simulink model "pyle_tf"  (R2020a)
settings: Solver=VariableStepAuto  StartTime=0.0  StopTime=0.2  RelTol=1e-3
libraries: fl_lib x71, nesl_utility x17, simulink x5, powerlib_meascontrol x1, ee_lib x1
(part 2 of 2)

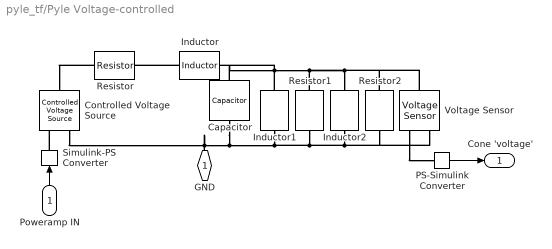
== system pyle_tf/Pyle Voltage-controlled ==
  Poweramp IN : Inport
  Capacitor : fl_lib/Electrical/Electrical Elements/Capacitor  c=388.95 uF  r=0 Ohm  g=0 1/Ohm  i_specify=off  i_priority=None  i=0 A  i_nominal_specify=off  i_nominal_unit=A  i_nominal_value=1  v_specify=off  v_priority=None  v=0 V  v_nominal_specify=off  v_nominal_unit=V  v_nominal_value=1  vc_specify=off  vc_priority=High  vc=0 V  vc_nominal_specify=off  vc_nominal_unit=V  vc_nominal_value=1
  Controlled Voltage Source : fl_lib/Electrical/Electrical Sources/Controlled Voltage Source
  Inductor : fl_lib/Electrical/Electrical Elements/Inductor  l=148.8 uH  r=0 Ohm  g=0 1/Ohm  i_specify=off  i_priority=None  i=0 A  i_nominal_specify=off  i_nominal_unit=A  i_nominal_value=1  v_specify=off  v_priority=None  v=0 V  v_nominal_specify=off  v_nominal_unit=V  v_nominal_value=1  i_L_specify=off  i_L_priority=High  i_L=0 A  i_L_nominal_specify=off  i_L_nominal_unit=A  i_L_nominal_value=1
  Inductor1 : fl_lib/Electrical/Electrical Elements/Inductor  l=23.9 mH  r=0 Ohm  g=0 1/Ohm  i_specify=off  i_priority=None  i=0 A  i_nominal_specify=off  i_nominal_unit=A  i_nominal_value=1  v_specify=off  v_priority=None  v=0 V  v_nominal_specify=off  v_nominal_unit=V  v_nominal_value=1  i_L_specify=off  i_L_priority=High  i_L=0 A  i_L_nominal_specify=off  i_L_nominal_unit=A  i_L_nominal_value=1
  Inductor2 : fl_lib/Electrical/Electrical Elements/Inductor  l=9 mH  r=0 Ohm  g=0 1/Ohm  i_specify=off  i_priority=None  i=0 A  i_nominal_specify=off  i_nominal_unit=A  i_nominal_value=1  v_specify=off  v_priority=None  v=0 V  v_nominal_specify=off  v_nominal_unit=V  v_nominal_value=1  i_L_specify=off  i_L_priority=High  i_L=0 A  i_L_nominal_specify=off  i_L_nominal_unit=A  i_L_nominal_value=1
  PS-Simulink Converter : nesl_utility/PS-Simulink Converter  PhysicalDomain=network_engine_domain  SubClassName=ps_output  LeftPortType=input  RightPortType=output  PseudoPeriodic=off  Frequencies=[]  Unit=inherit  AffineConversion=off
  Resistor : fl_lib/Electrical/Electrical Elements/Resistor  R=3.4 Ohm  i_specify=off  i_priority=None  i=0 A  i_nominal_specify=off  i_nominal_unit=A  i_nominal_value=1  v_specify=off  v_priority=None  v=0 V  v_nominal_specify=off  v_nominal_unit=V  v_nominal_value=1
  Resistor1 : fl_lib/Electrical/Electrical Elements/Resistor  R=28.42 Ohm  i_specify=off  i_priority=None  i=0 A  i_nominal_specify=off  i_nominal_unit=A  i_nominal_value=1  v_specify=off  v_priority=None  v=0 V  v_nominal_specify=off  v_nominal_unit=V  v_nominal_value=1
  Resistor2 : fl_lib/Electrical/Electrical Elements/Resistor  R=282 Ohm  i_specify=off  i_priority=None  i=0 A  i_nominal_specify=off  i_nominal_unit=A  i_nominal_value=1  v_specify=off  v_priority=None  v=0 V  v_nominal_specify=off  v_nominal_unit=V  v_nominal_value=1
  Simulink-PS Converter : nesl_utility/Simulink-PS Converter  PhysicalDomain=network_engine_domain  SubClassName=ps_input  LeftPortType=input  RightPortType=output  PseudoPeriodic=off  Frequencies=[]  NoiseDistribution=none  NoiseParameters=[]  Unit=1  AffineConversion=off  FilteringAndDerivatives=provide  SimscapeFilterOrder=1  InputFilterTimeConstant=0.001  UdotUserProvided=0
  Voltage Sensor : fl_lib/Electrical/Electrical Sensors/Voltage Sensor
  GND : PMIOPort  Side=Right
  Cone 'voltage' : Outport
  wires:
  PS-Simulink Converter/1 -> Cone 'voltage'/1
  Poweramp IN/1 -> Simulink-PS Converter/1
  connections:
  Voltage Sensor/RConn1 -- PS-Simulink Converter/LConn1
  Simulink-PS Converter/RConn1 -- Controlled Voltage Source/RConn1
  Controlled Voltage Source/RConn2 -- GND/RConn1 -- Resistor2/RConn1 -- Voltage Sensor/RConn2 -- Inductor2/RConn1 -- Resistor1/RConn1 -- Inductor1/RConn1 -- Capacitor/RConn1
  Inductor1/LConn1 -- Inductor2/LConn1 -- Voltage Sensor/LConn1 -- Resistor2/LConn1 -- Resistor1/LConn1 -- Capacitor/LConn1 -- Inductor/RConn1
  Inductor/LConn1 -- Resistor/RConn1
  Resistor/LConn1 -- Controlled Voltage Source/LConn1

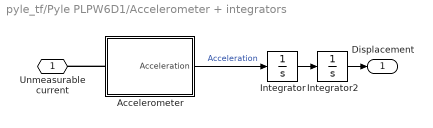
== system pyle_tf/Pyle PLPW6D1/Accelerometer + integrators ==
  Accelerometer : Subsystem
  Integrator : Integrator
  Integrator2 : Integrator
  Unmeasurable current : PMIOPort  Side=Left
  Displacement : Outport
  wires:
  Integrator2/1 -> Displacement/1
  Integrator/1 -> Integrator2/1
  Accelerometer/1(Acceleration) -> Integrator/1  "Acceleration"
  connections:
  Accelerometer/LConn1 -- Unmeasurable current/RConn1

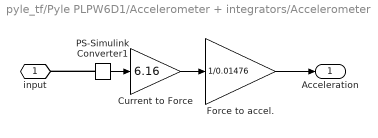
== system pyle_tf/Pyle PLPW6D1/Accelerometer + integrators/Accelerometer ==
  Current to Force : Gain  Gain=6.16
  Force to accel. : Gain  Gain=1/0.01476
  PS-Simulink Converter1 : nesl_utility/PS-Simulink Converter  PhysicalDomain=network_engine_domain  SubClassName=ps_output  LeftPortType=input  RightPortType=output  PseudoPeriodic=off  Frequencies=[]  Unit=inherit  AffineConversion=off
  input : PMIOPort  Side=Left
  Acceleration : Outport
  wires:
  Force to accel./1 -> Acceleration/1
  Current to Force/1 -> Force to accel./1
  PS-Simulink Converter1/1 -> Current to Force/1
  connections:
  PS-Simulink Converter1/LConn1 -- input/RConn1
